simulink model "Kronauer_Model_Paper"  (R2015a)
settings: Solver=ode3  StartTime=0.0  StopTime=450  FixedStep=0.01  MaxStep=0.01  RelTol=1e-5
values from neighbouring files (symbols this model uses):
  Imax = 1000    [Gradient_Descent_Greedy_3rd.m]
  n0 = Periodic_Solution(time_shift(j)*100+1,4)    [Gradient_Descent_Greedy_3rd.m]
  Periodic_Solution = Periodic_Solution(101:end,:)    [Gradient_Descent_Greedy_3rd.m]    (also in Periodic_Solution_JFK_1000lux.mat = [0 0.00999999999999 0.02 0.03 0.04 0.05 0.0599999999999 0.06)
  tol = 0.01    [Gradient_Descent_Greedy_3rd.m]
  x0 = Periodic_Solution(time_shift(j)*100+1,2)    [Gradient_Descent_Greedy_3rd.m]
  xc0 = Periodic_Solution(time_shift(j)*100+1,3)    [Gradient_Descent_Greedy_3rd.m]
undefined symbols (not defined in the file or in its folder): I
settings Model: Creator=Zhang Jiaxiang  LastModifiedBy=Jiawei Yin
settings DataIOCC: LimitDataPoints=off  SignalLoggingSaveFormat=ModelDataLogs
settings OptimizationCC: ExpressionDepthLimit=2147483647
settings DebuggingCC: UnderspecifiedInitializationDetection=Classic  MergeDetectMultiDrivingBlocksExec=none  FcnCallInpInsideContextMsg=UseLocalSettings  StateNameClashWarn=warning
settings GRTTargetCC: CombineOutputUpdateFcns=off  GRTInterface=on

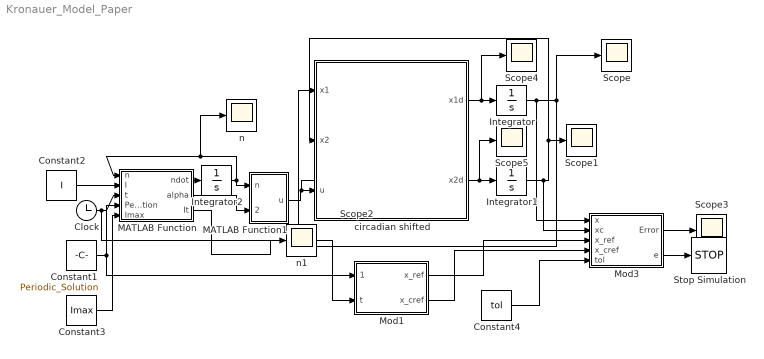
== system Kronauer_Model_Paper ==
  Clock : Clock
  Constant1 : Constant  Value=Periodic_Solution
  Constant2 : Constant  Value=I
  Constant3 : Constant  Value=Imax
  Constant4 : Constant  Value=tol
  Integrator : Integrator  InitialCondition=x0
  Integrator1 : Integrator  InitialCondition=xc0
  Integrator2 : Integrator  InitialCondition=n0
  MATLAB Function : MATLAB Function  TreatAsAtomicUnit=on
      settings: PermitHierarchicalResolution=ParametersOnly
  MATLAB Function1 : MATLAB Function  TreatAsAtomicUnit=on
      settings: PermitHierarchicalResolution=ParametersOnly
  Mod1 : MATLAB Function  TreatAsAtomicUnit=on
      settings: PermitHierarchicalResolution=ParametersOnly
  Mod3 : MATLAB Function  TreatAsAtomicUnit=on
      settings: PermitHierarchicalResolution=ParametersOnly
  Scope{,1..5} (6 alike) : Scope
      Scope settings: TimeRange=auto  LimitDataPoints=on  MaxDataPoints=1000000  SaveName=x  YMin=-1.15396  YMax=0.97021  SampleTime=-1  DataFormat=Array
      Scope1 settings: TimeRange=auto  LimitDataPoints=on  MaxDataPoints=1000000  SaveName=xc  YMin=-1.29085  YMax=0.80259  SampleTime=-1  DataFormat=Array
      Scope2 settings: TimeRange=auto  LimitDataPoints=on  MaxDataPoints=1000000  SaveName=u  YMin=-10  YMax=10  SampleTime=-1  DataFormat=Array
      Scope3 settings: TimeRange=auto  LimitDataPoints=on  MaxDataPoints=100000000  SaveName=Error  YMin=-10  YMax=10  SampleTime=-1  DataFormat=Array
      Scope4 settings: TimeRange=auto  LimitDataPoints=on  MaxDataPoints=1000000  SaveName=dx  YMin=-0.38511  YMax=0.63191  SampleTime=-1  DataFormat=Array
      Scope5 settings: TimeRange=auto  LimitDataPoints=on  MaxDataPoints=1000000  SaveName=dxc  YMin=-0.25827  YMax=0.34342  SampleTime=-1  DataFormat=Array
  Stop Simulation : Stop
  circadian shifted : MATLAB Function  TreatAsAtomicUnit=on
      settings: PermitHierarchicalResolution=ParametersOnly
  n : Scope
      settings: TimeRange=auto  LimitDataPoints=on  MaxDataPoints=2000000  SaveName=n  YMin=-10  YMax=10  SampleTime=-1  DataFormat=Array
  n1 : Scope
      settings: TimeRange=auto  LimitDataPoints=on  MaxDataPoints=200000000  SaveName=It  YMin=-10  YMax=10  SampleTime=-1  DataFormat=Array
  wires:
  circadian shifted/1(x1d) -> Scope4/1, Integrator/1
  circadian shifted/2(x2d) -> Scope5/1, Integrator1/1
  Integrator/1 -> Mod3/1(x), circadian shifted/1(x1), Scope/1
  Integrator1/1 -> Mod3/2(xc), circadian shifted/2(x2), Scope1/1
  MATLAB Function/1(ndot) -> Integrator2/1
  Constant2/1 -> MATLAB Function/2(I)
  Clock/1 -> Mod1/2(t), MATLAB Function/3(t)
  Integrator2/1 -> MATLAB Function1/1(n), n/1, MATLAB Function/1(n)
  MATLAB Function/2(alpha) -> MATLAB Function1/2(alpha)
  MATLAB Function1/1(u) -> Scope2/1, circadian shifted/3(u)
  Constant1/1 -> MATLAB Function/4(Periodic_Solution), Mod1/1(Periodic_Solution)
  Constant3/1 -> MATLAB Function/5(Imax)
  Mod3/2(e) -> Stop Simulation/1
  Constant4/1 -> Mod3/5(tol)
  Mod1/1(x_ref) -> Mod3/3(x_ref)
  Mod1/2(x_cref) -> Mod3/4(x_cref)
  Mod3/1(Error) -> Scope3/1
  MATLAB Function/3(It) -> n1/1

== matlab function Kronauer_Model_Paper/circadian shifted ==
  data: x1 input; x2 input; u input; x1d output; x2d output
function [ x1d,x2d] = fcn(x1,x2,u)
%#eml

q = 1/3;
taux = 24.2;
k = 0.55;
mu=0.13;

B = u*(1-0.4*x1)*(1-0.4*x2);

x1d = (pi/12)*(x2 + B  + mu*(1/3*x1 + 4/3*x1^3 - 256/105*x1^7));
x2d = (pi/12)*(q*B *x2 - (24/(taux*0.99729))^2*x1 - k*B*x1);

== matlab function Kronauer_Model_Paper/MATLAB Function ==
  data: n input; I input; ndot output; t input; alpha output; Periodic_Solution input; Imax input; It output
function [ndot,alpha,It] = fcn(n,I,t,Periodic_Solution,Imax)

alpha0=0.05;
beta=0.0075;
I0=9500;
if t<I(end,1)
    It=interp1q(I(:,1),I(:,2),t);
else
    It=interp1q(Periodic_Solution(:,1),Periodic_Solution(:,4),t);
    if It~=0
        It=Imax;
    end
end
alpha=alpha0*(It/I0)^0.5;
ndot=60*[alpha*(1-n)-beta*n];

== matlab function Kronauer_Model_Paper/MATLAB Function1 ==
  data: n input; u output; alpha input
function u = fcn(n,alpha)
%#codegen
u=33.75*alpha*(1-n);

== matlab function Kronauer_Model_Paper/Mod1 ==
  data: Periodic_Solution input; x_ref output; t input; x_cref output
function [x_ref,x_cref] = fcn(Periodic_Solution,t)
%#codegen
x_ref=interp1q(Periodic_Solution(:,1),Periodic_Solution(:,2),t);
x_cref=interp1q(Periodic_Solution(:,1),Periodic_Solution(:,3),t);

== matlab function Kronauer_Model_Paper/Mod3 ==
  data: Error output; x input; xc input; e output; x_ref input; x_cref input; tol input
function [Error,e] = fcn(x,xc,x_ref,x_cref,tol)
%#codegen
Error=(x-x_ref)^2+(xc-x_cref)^2;
e=Error<tol;
